simulink library "controllers"  (R2018a)
settings: Solver=VariableStepAuto  StartTime=0.0  StopTime=10.0  RelTol=1e-3
undefined symbols (not defined in the file): ctrl, plant
libraries: controllerComponents x24, simulink x14
settings Model: Creator=mitch  LastModifiedBy=mitch

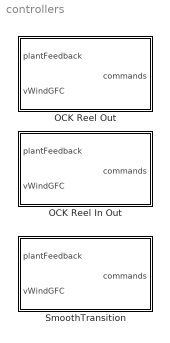
== system controllers ==
  OCK Reel In Out : Subsystem  VariantControl=variantOCKReelInOut
  OCK Reel Out : Subsystem  VariantControl=variantOCK
  SmoothTransition : Subsystem  VariantControl=variantOCKReelInOut

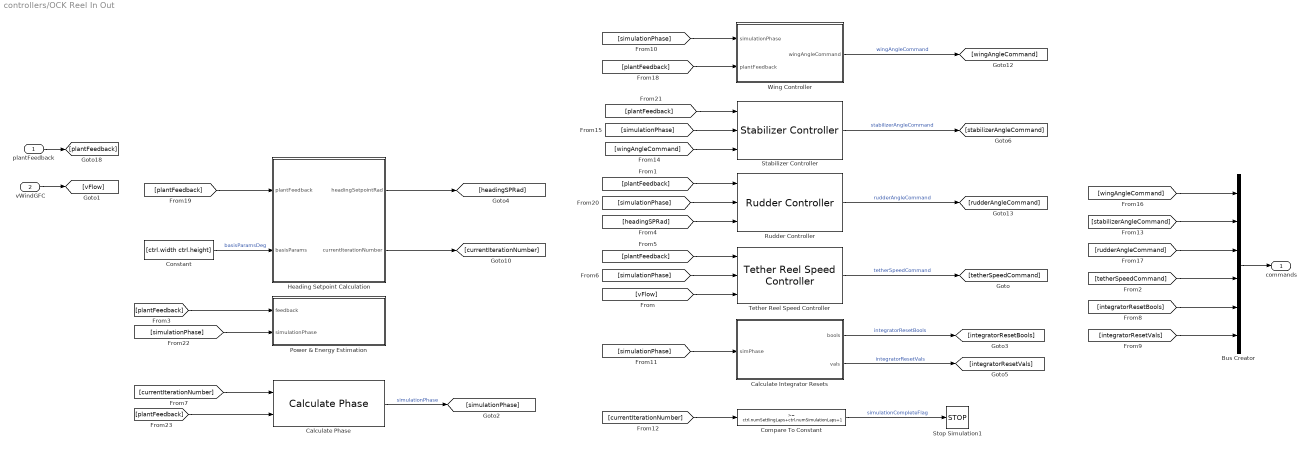
== system controllers/OCK Reel In Out ==
  plantFeedback : Inport  OutDataTypeStr=Bus: busPlantFeedback
  vWindGFC : Inport  Port=2
  Bus Creator : BusCreator  Inputs=6  OutDataTypeStr=Bus: busControllerOutput
  Calculate Integrator Resets : Subsystem
  Calculate Phase : controllerComponents/Calculate Phase
  Compare To Constant : simulink/Logic and Bit Operations/Compare To Constant  relop=>=  const=ctrl.numSettlingLaps+ctrl.numSimulationLaps+1  OutDataTypeStr=boolean
  Constant : Constant  Value=[ctrl.width ctrl.height]
  Heading Setpoint Calculation : Subsystem  VariantControl=variantPureCarrotFollowing
  Power & Energy Estimation : Subsystem
  Rudder Controller : controllerComponents/Rudder Controller
  Stabilizer Controller : controllerComponents/Stabilizer Controller
  Stop Simulation1 : Stop
  Tether Reel Speed Controller : controllerComponents/Tether Reel Speed Controller
  Wing Controller : Subsystem
  commands : Outport  OutDataTypeStr=Bus: busControllerOutput
  wires:
  [plantFeedback] -> Heading Setpoint Calculation/1(plantFeedback)
  Constant/1 -> Heading Setpoint Calculation/2(basisParams)  "basisParamsDeg"
  plantFeedback/1 -> [plantFeedback]
  vWindGFC/1 -> [vFlow]
  Bus Creator/1 -> commands/1
  [currentIterationNumber] -> Compare To Constant/1
  Compare To Constant/1 -> Stop Simulation1/1  "simulationCompleteFlag"
  Heading Setpoint Calculation/2(currentIterationNumber) -> [currentIterationNumber]
  Heading Setpoint Calculation/1(headingSetpointRad) -> [headingSPRad]
  Rudder Controller/1 -> [rudderAngleCommand]  "rudderAngleCommand"
  Tether Reel Speed Controller/1 -> [tetherSpeedCommand]  "tetherSpeedCommand"
  [plantFeedback] -> Power & Energy Estimation/1(feedback)
  [currentIterationNumber] -> Calculate Phase/1
  Calculate Phase/1 -> [simulationPhase]  "simulationPhase"
  [plantFeedback] -> Wing Controller/2(plantFeedback)
  Wing Controller/1(wingAngleCommand) -> [wingAngleCommand]  "wingAngleCommand"
  [simulationPhase] -> Wing Controller/1(simulationPhase)
  [simulationPhase] -> Calculate Integrator Resets/1(simPhase)
  Calculate Integrator Resets/1(bools) -> [integratorResetBools]  "integratorResetBools"
  Calculate Integrator Resets/2(vals) -> [integratorResetVals]  "integratorResetVals"
  [vFlow] -> Tether Reel Speed Controller/3
  [plantFeedback] -> Tether Reel Speed Controller/1
  [simulationPhase] -> Tether Reel Speed Controller/2
  [integratorResetVals] -> Bus Creator/6
  [integratorResetBools] -> Bus Creator/5
  [tetherSpeedCommand] -> Bus Creator/4
  [rudderAngleCommand] -> Bus Creator/3
  [wingAngleCommand] -> Bus Creator/1
  Stabilizer Controller/1 -> [stabilizerAngleCommand]  "stabilizerAngleCommand"
  [stabilizerAngleCommand] -> Bus Creator/2
  [plantFeedback] -> Rudder Controller/1
  [headingSPRad] -> Rudder Controller/3
  [simulationPhase] -> Rudder Controller/2
  [simulationPhase] -> Stabilizer Controller/2
  [plantFeedback] -> Stabilizer Controller/1
  [wingAngleCommand] -> Stabilizer Controller/3
  [simulationPhase] -> Power & Energy Estimation/2(simulationPhase)
  [plantFeedback] -> Calculate Phase/2

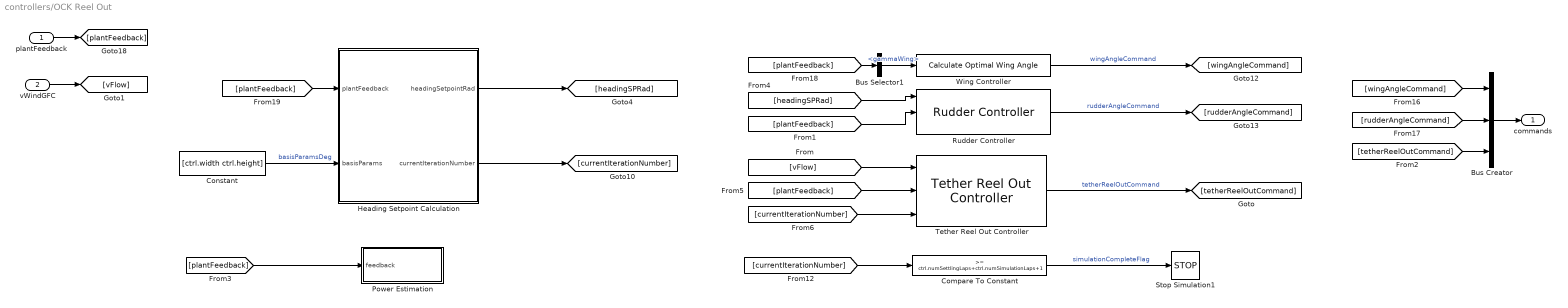
== system controllers/OCK Reel Out ==
  plantFeedback : Inport  OutDataTypeStr=Bus: busPlantFeedback
  vWindGFC : Inport  Port=2
  Bus Creator : BusCreator  Inputs=3  OutDataTypeStr=Bus: busControllerOutput
  Bus Selector1 : BusSelector  OutputSignals=gammaWing
  Compare To Constant : simulink/Logic and Bit Operations/Compare To Constant  relop=>=  const=ctrl.numSettlingLaps+ctrl.numSimulationLaps+1  OutDataTypeStr=boolean
  Constant : Constant  Value=[ctrl.width ctrl.height]
  Heading Setpoint Calculation : Subsystem  VariantControl=variantPureCarrotFollowing
  Power Estimation : Subsystem
  Rudder Controller : controllerComponents/Rudder Controller
  Stop Simulation1 : Stop
  Tether Reel Out Controller : controllerComponents/Tether Reel Out Controller
  Wing Controller : controllerComponents/Calculate Optimal Wing Angle
  commands : Outport  OutDataTypeStr=Bus: busControllerOutput
  wires:
  [plantFeedback] -> Heading Setpoint Calculation/1(plantFeedback)
  Constant/1 -> Heading Setpoint Calculation/2(basisParams)  "basisParamsDeg"
  [plantFeedback] -> Rudder Controller/2
  [plantFeedback] -> Bus Selector1/1
  plantFeedback/1 -> [plantFeedback]
  vWindGFC/1 -> [vFlow]
  Bus Selector1/1 -> Wing Controller/1  "<gammaWing>"
  Bus Creator/1 -> commands/1
  [rudderAngleCommand] -> Bus Creator/2
  [wingAngleCommand] -> Bus Creator/1
  [currentIterationNumber] -> Compare To Constant/1
  Compare To Constant/1 -> Stop Simulation1/1  "simulationCompleteFlag"
  Heading Setpoint Calculation/2(currentIterationNumber) -> [currentIterationNumber]
  Heading Setpoint Calculation/1(headingSetpointRad) -> [headingSPRad]
  [headingSPRad] -> Rudder Controller/1
  Rudder Controller/1 -> [rudderAngleCommand]  "rudderAngleCommand"
  Wing Controller/1 -> [wingAngleCommand]  "wingAngleCommand"
  [tetherReelOutCommand] -> Bus Creator/3
  Tether Reel Out Controller/1 -> [tetherReelOutCommand]  "tetherReelOutCommand"
  [vFlow] -> Tether Reel Out Controller/1
  [plantFeedback] -> Power Estimation/1(feedback)
  [plantFeedback] -> Tether Reel Out Controller/2
  [currentIterationNumber] -> Tether Reel Out Controller/3

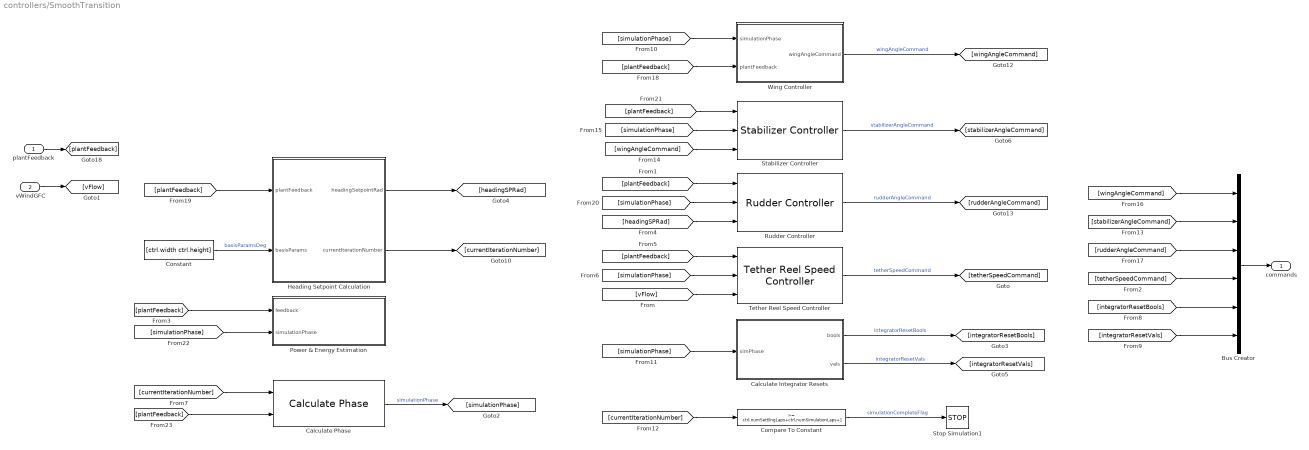
== system controllers/SmoothTransition ==
  plantFeedback : Inport  OutDataTypeStr=Bus: busPlantFeedback
  vWindGFC : Inport  Port=2
  Bus Creator : BusCreator  Inputs=6  OutDataTypeStr=Bus: busControllerOutput
  Calculate Integrator Resets : Subsystem
  Calculate Phase : controllerComponents/Calculate Phase
  Compare To Constant : simulink/Logic and Bit Operations/Compare To Constant  relop=>=  const=ctrl.numSettlingLaps+ctrl.numSimulationLaps+1  OutDataTypeStr=boolean
  Constant : Constant  Value=[ctrl.width ctrl.height]
  Heading Setpoint Calculation : Subsystem  VariantControl=variantPureCarrotFollowing
  Power & Energy Estimation : Subsystem
  Rudder Controller : controllerComponents/Rudder Controller
  Stabilizer Controller : controllerComponents/Stabilizer Controller
  Stop Simulation1 : Stop
  Tether Reel Speed Controller : controllerComponents/Tether Reel Speed Controller
  Wing Controller : Subsystem
  commands : Outport  OutDataTypeStr=Bus: busControllerOutput
  wires:
  [plantFeedback] -> Heading Setpoint Calculation/1(plantFeedback)
  Constant/1 -> Heading Setpoint Calculation/2(basisParams)  "basisParamsDeg"
  plantFeedback/1 -> [plantFeedback]
  vWindGFC/1 -> [vFlow]
  Bus Creator/1 -> commands/1
  [currentIterationNumber] -> Compare To Constant/1
  Compare To Constant/1 -> Stop Simulation1/1  "simulationCompleteFlag"
  Heading Setpoint Calculation/2(currentIterationNumber) -> [currentIterationNumber]
  Heading Setpoint Calculation/1(headingSetpointRad) -> [headingSPRad]
  Rudder Controller/1 -> [rudderAngleCommand]  "rudderAngleCommand"
  Tether Reel Speed Controller/1 -> [tetherSpeedCommand]  "tetherSpeedCommand"
  [plantFeedback] -> Power & Energy Estimation/1(feedback)
  [currentIterationNumber] -> Calculate Phase/1
  Calculate Phase/1 -> [simulationPhase]  "simulationPhase"
  [plantFeedback] -> Wing Controller/2(plantFeedback)
  Wing Controller/1(wingAngleCommand) -> [wingAngleCommand]  "wingAngleCommand"
  [simulationPhase] -> Wing Controller/1(simulationPhase)
  [simulationPhase] -> Calculate Integrator Resets/1(simPhase)
  Calculate Integrator Resets/1(bools) -> [integratorResetBools]  "integratorResetBools"
  Calculate Integrator Resets/2(vals) -> [integratorResetVals]  "integratorResetVals"
  [vFlow] -> Tether Reel Speed Controller/3
  [plantFeedback] -> Tether Reel Speed Controller/1
  [simulationPhase] -> Tether Reel Speed Controller/2
  [integratorResetVals] -> Bus Creator/6
  [integratorResetBools] -> Bus Creator/5
  [tetherSpeedCommand] -> Bus Creator/4
  [rudderAngleCommand] -> Bus Creator/3
  [wingAngleCommand] -> Bus Creator/1
  Stabilizer Controller/1 -> [stabilizerAngleCommand]  "stabilizerAngleCommand"
  [stabilizerAngleCommand] -> Bus Creator/2
  [plantFeedback] -> Rudder Controller/1
  [headingSPRad] -> Rudder Controller/3
  [simulationPhase] -> Rudder Controller/2
  [simulationPhase] -> Stabilizer Controller/2
  [plantFeedback] -> Stabilizer Controller/1
  [wingAngleCommand] -> Stabilizer Controller/3
  [simulationPhase] -> Power & Energy Estimation/2(simulationPhase)
  [plantFeedback] -> Calculate Phase/2

== system controllers/OCK Reel In Out/Calculate Integrator Resets ==
  simPhase : Inport
  Calculate Booleans : Subsystem
  Calculate Values : Subsystem
  Compare To Constant : simulink/Logic and Bit Operations/Compare To Constant  relop===  const=2  OutDataTypeStr=boolean
  Delay : Delay  DelayLength=1  InitialCondition=0
  bools : Outport
  vals : Outport  Port=2
  wires:
  simPhase/1 -> Delay/1
  Calculate Booleans/1(bools) -> bools/1
  Calculate Values/1(bools) -> vals/1
  Compare To Constant/1 -> Calculate Booleans/1(reelInFlag), Calculate Values/1(reelInFlag)
  Delay/1 -> Compare To Constant/1

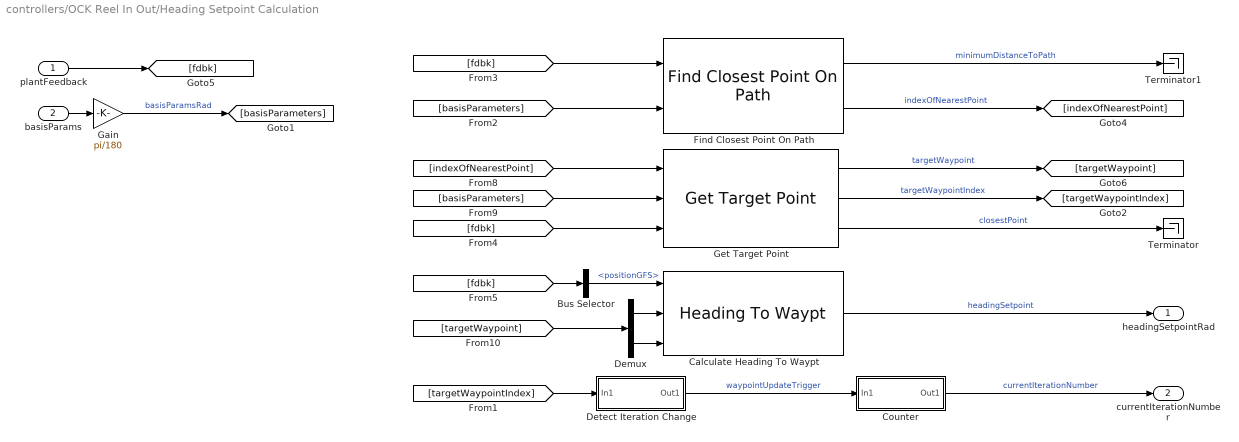
== system controllers/OCK Reel In Out/Heading Setpoint Calculation ==
  plantFeedback : Inport  OutDataTypeStr=Bus: busPlantFeedback
  basisParams : Inport  Port=2
  Bus Selector : BusSelector  OutputSignals=positionGFS
  Calculate Heading To Waypt : controllerComponents/Heading To Waypt
  Counter : Subsystem
  Demux : Demux  Outputs=2
  Detect Iteration Change : Subsystem
  Find Closest Point On Path : controllerComponents/Find Closest Point On Path
  Gain : Gain  Gain=pi/180
  Get Target Point : controllerComponents/Get Target Point
  Terminator : Terminator
  Terminator1 : Terminator
  headingSetpointRad : Outport
  currentIterationNumber : Outport  Port=2
  wires:
  Get Target Point/3 -> Terminator/1  "closestPoint"
  plantFeedback/1 -> [fdbk]
  Get Target Point/2 -> [targetWaypointIndex]  "targetWaypointIndex"
  Detect Iteration Change/1(Out1) -> Counter/1(In1)  "waypointUpdateTrigger"
  Counter/1(Out1) -> currentIterationNumber/1  "currentIterationNumber"
  [targetWaypointIndex] -> Detect Iteration Change/1(In1)
  Calculate Heading To Waypt/1 -> headingSetpointRad/1  "headingSetpoint"
  [targetWaypoint] -> Demux/1
  Get Target Point/1 -> [targetWaypoint]  "targetWaypoint"
  [basisParameters] -> Get Target Point/2
  [indexOfNearestPoint] -> Get Target Point/1
  Find Closest Point On Path/2 -> [indexOfNearestPoint]  "indexOfNearestPoint"
  Find Closest Point On Path/1 -> Terminator1/1  "minimumDistanceToPath"
  Demux/2 -> Calculate Heading To Waypt/3
  Demux/1 -> Calculate Heading To Waypt/2
  [basisParameters] -> Find Closest Point On Path/2
  [fdbk] -> Find Closest Point On Path/1
  [fdbk] -> Get Target Point/3
  basisParams/1 -> Gain/1
  [fdbk] -> Bus Selector/1
  Bus Selector/1 -> Calculate Heading To Waypt/1  "<positionGFS>"
  Gain/1 -> [basisParameters]  "basisParamsRad"

== system controllers/OCK Reel In Out/Power & Energy Estimation ==
  feedback : Inport
  simulationPhase : Inport  Port=2
  Bus Selector : BusSelector  OutputSignals=rDot,tetherTension
  Compare To Constant : simulink/Logic and Bit Operations/Compare To Constant  relop=>=  const=1  OutDataTypeStr=boolean
  Constant : Constant  Value=0
  Integrator : Integrator  ExternalReset=rising  InitialConditionSource=external
  Product : Product
  Terminator : Terminator
  Terminator1 : Terminator
  wires:
  Product/1 -> Integrator/1, Terminator/1  "powerEstimate"
  feedback/1 -> Bus Selector/1
  Bus Selector/1 -> Product/1  "<rDot>"
  Bus Selector/2 -> Product/2  "<tetherTension>"
  Integrator/1 -> Terminator1/1  "netEnergy"
  simulationPhase/1 -> Compare To Constant/1
  Compare To Constant/1 -> Integrator/2
  Constant/1 -> Integrator/3

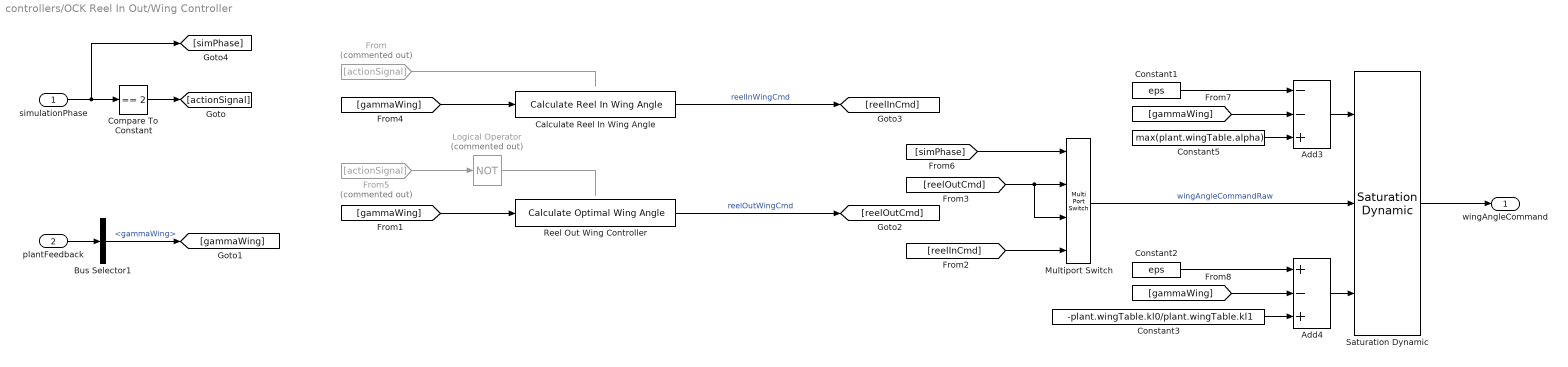
== system controllers/OCK Reel In Out/Wing Controller ==
  simulationPhase : Inport
  plantFeedback : Inport  Port=2
  Add3 : Sum  Inputs=--+
  Add4 : Sum  Inputs=+-+
  Bus Selector1 : BusSelector  OutputSignals=gammaWing
  Calculate Reel In Wing Angle : controllerComponents/Calculate Reel In Wing Angle
  Compare To Constant : simulink/Logic and Bit Operations/Compare To Constant  relop===  const=2  OutDataTypeStr=boolean
  Constant1 : Constant  Value=eps
  Constant2 : Constant  Value=eps
  Constant3 : Constant  Value=-plant.wingTable.kl0/plant.wingTable.kl1
  Constant5 : Constant  Value=max(plant.wingTable.alpha)
  From : From  Commented=on  GotoTag=actionSignal
  From5 : From  Commented=on  GotoTag=actionSignal
  Logical Operator : Logic  Commented=on  Operator=NOT  AllPortsSameDT=off  OutDataTypeStr=boolean
  Multiport Switch : MultiPortSwitch  DataPortOrder=Zero-based contiguous  zeroidx=on
  Reel Out Wing Controller : controllerComponents/Calculate Optimal Wing Angle
  Saturation Dynamic : simulink/Discontinuities/Saturation Dynamic  OutMin=[]  OutMax=[]  OutDataTypeStr=Inherit: Same as second input  OutDataType=fixdt(1, 16)  OutScaling=2^-10  DoSatur=off
  wingAngleCommand : Outport
  wires:
  plantFeedback/1 -> Bus Selector1/1
  simulationPhase/1 -> [simPhase], Compare To Constant/1
  Add4/1 -> Saturation Dynamic/3
  Add3/1 -> Saturation Dynamic/1
  Saturation Dynamic/1 -> wingAngleCommand/1
  Bus Selector1/1 -> [gammaWing]  "<gammaWing>"
  [gammaWing] -> Reel Out Wing Controller/1
  Reel Out Wing Controller/1 -> [reelOutCmd]  "reelOutWingCmd"
  Calculate Reel In Wing Angle/1 -> [reelInCmd]  "reelInWingCmd"
  [gammaWing] -> Calculate Reel In Wing Angle/1
  Logical Operator/1 -> ?
  Compare To Constant/1 -> [actionSignal]
  From/1 -> ?
  From5/1 -> Logical Operator/1
  Constant5/1 -> Add3/3
  Constant1/1 -> Add3/1
  [gammaWing] -> Add3/2
  Constant3/1 -> Add4/3
  [gammaWing] -> Add4/2
  Constant2/1 -> Add4/1
  Multiport Switch/1 -> Saturation Dynamic/2  "wingAngleCommandRaw"
  [simPhase] -> Multiport Switch/1
  [reelOutCmd] -> Multiport Switch/3, Multiport Switch/2
  [reelInCmd] -> Multiport Switch/4

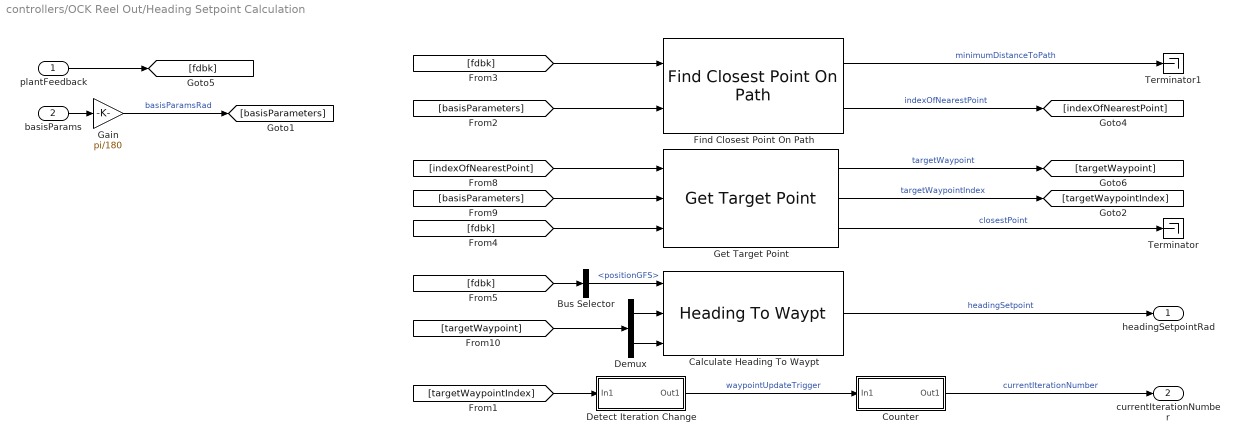
== system controllers/OCK Reel Out/Heading Setpoint Calculation ==
  plantFeedback : Inport  OutDataTypeStr=Bus: busPlantFeedback
  basisParams : Inport  Port=2
  Bus Selector : BusSelector  OutputSignals=positionGFS
  Calculate Heading To Waypt : controllerComponents/Heading To Waypt
  Counter : Subsystem
  Demux : Demux  Outputs=2
  Detect Iteration Change : Subsystem
  Find Closest Point On Path : controllerComponents/Find Closest Point On Path
  Gain : Gain  Gain=pi/180
  Get Target Point : controllerComponents/Get Target Point
  Terminator : Terminator
  Terminator1 : Terminator
  headingSetpointRad : Outport
  currentIterationNumber : Outport  Port=2
  wires:
  Get Target Point/3 -> Terminator/1  "closestPoint"
  plantFeedback/1 -> [fdbk]
  Get Target Point/2 -> [targetWaypointIndex]  "targetWaypointIndex"
  Detect Iteration Change/1(Out1) -> Counter/1(In1)  "waypointUpdateTrigger"
  Counter/1(Out1) -> currentIterationNumber/1  "currentIterationNumber"
  [targetWaypointIndex] -> Detect Iteration Change/1(In1)
  Calculate Heading To Waypt/1 -> headingSetpointRad/1  "headingSetpoint"
  [targetWaypoint] -> Demux/1
  Get Target Point/1 -> [targetWaypoint]  "targetWaypoint"
  [basisParameters] -> Get Target Point/2
  [indexOfNearestPoint] -> Get Target Point/1
  Find Closest Point On Path/2 -> [indexOfNearestPoint]  "indexOfNearestPoint"
  Find Closest Point On Path/1 -> Terminator1/1  "minimumDistanceToPath"
  Demux/2 -> Calculate Heading To Waypt/3
  Demux/1 -> Calculate Heading To Waypt/2
  [basisParameters] -> Find Closest Point On Path/2
  [fdbk] -> Find Closest Point On Path/1
  [fdbk] -> Get Target Point/3
  basisParams/1 -> Gain/1
  [fdbk] -> Bus Selector/1
  Bus Selector/1 -> Calculate Heading To Waypt/1  "<positionGFS>"
  Gain/1 -> [basisParameters]  "basisParamsRad"

== system controllers/OCK Reel Out/Power Estimation ==
  feedback : Inport
  Bus Selector : BusSelector  OutputSignals=rDot,tetherTension
  Product : Product
  Terminator : Terminator
  wires:
  Product/1 -> Terminator/1  "powerEstimate"
  feedback/1 -> Bus Selector/1
  Bus Selector/1 -> Product/1  "<rDot>"
  Bus Selector/2 -> Product/2  "<tetherTension>"

== system controllers/SmoothTransition/Calculate Integrator Resets ==
  simPhase : Inport
  Calculate Booleans : Subsystem
  Calculate Values : Subsystem
  Compare To Constant : simulink/Logic and Bit Operations/Compare To Constant  relop===  const=2  OutDataTypeStr=boolean
  Delay : Delay  DelayLength=1  InitialCondition=0
  bools : Outport
  vals : Outport  Port=2
  wires:
  simPhase/1 -> Delay/1
  Calculate Booleans/1(bools) -> bools/1
  Calculate Values/1(bools) -> vals/1
  Compare To Constant/1 -> Calculate Booleans/1(reelInFlag), Calculate Values/1(reelInFlag)
  Delay/1 -> Compare To Constant/1

== system controllers/SmoothTransition/Heading Setpoint Calculation ==
  plantFeedback : Inport  OutDataTypeStr=Bus: busPlantFeedback
  basisParams : Inport  Port=2
  Bus Selector : BusSelector  OutputSignals=positionGFS
  Calculate Heading To Waypt : controllerComponents/Heading To Waypt
  Counter : Subsystem
  Demux : Demux  Outputs=2
  Detect Iteration Change : Subsystem
  Find Closest Point On Path : controllerComponents/Find Closest Point On Path
  Gain : Gain  Gain=pi/180
  Get Target Point : controllerComponents/Get Target Point
  Terminator : Terminator
  Terminator1 : Terminator
  headingSetpointRad : Outport
  currentIterationNumber : Outport  Port=2
  wires:
  Get Target Point/3 -> Terminator/1  "closestPoint"
  plantFeedback/1 -> [fdbk]
  Get Target Point/2 -> [targetWaypointIndex]  "targetWaypointIndex"
  Detect Iteration Change/1(Out1) -> Counter/1(In1)  "waypointUpdateTrigger"
  Counter/1(Out1) -> currentIterationNumber/1  "currentIterationNumber"
  [targetWaypointIndex] -> Detect Iteration Change/1(In1)
  Calculate Heading To Waypt/1 -> headingSetpointRad/1  "headingSetpoint"
  [targetWaypoint] -> Demux/1
  Get Target Point/1 -> [targetWaypoint]  "targetWaypoint"
  [basisParameters] -> Get Target Point/2
  [indexOfNearestPoint] -> Get Target Point/1
  Find Closest Point On Path/2 -> [indexOfNearestPoint]  "indexOfNearestPoint"
  Find Closest Point On Path/1 -> Terminator1/1  "minimumDistanceToPath"
  Demux/2 -> Calculate Heading To Waypt/3
  Demux/1 -> Calculate Heading To Waypt/2
  [basisParameters] -> Find Closest Point On Path/2
  [fdbk] -> Find Closest Point On Path/1
  [fdbk] -> Get Target Point/3
  basisParams/1 -> Gain/1
  [fdbk] -> Bus Selector/1
  Bus Selector/1 -> Calculate Heading To Waypt/1  "<positionGFS>"
  Gain/1 -> [basisParameters]  "basisParamsRad"

== system controllers/SmoothTransition/Power & Energy Estimation ==
  feedback : Inport
  simulationPhase : Inport  Port=2
  Bus Selector : BusSelector  OutputSignals=rDot,tetherTension
  Compare To Constant : simulink/Logic and Bit Operations/Compare To Constant  relop=>=  const=1  OutDataTypeStr=boolean
  Constant : Constant  Value=0
  Integrator : Integrator  ExternalReset=rising  InitialConditionSource=external
  Product : Product
  Terminator : Terminator
  Terminator1 : Terminator
  wires:
  Product/1 -> Integrator/1, Terminator/1  "powerEstimate"
  feedback/1 -> Bus Selector/1
  Bus Selector/1 -> Product/1  "<rDot>"
  Bus Selector/2 -> Product/2  "<tetherTension>"
  Integrator/1 -> Terminator1/1  "netEnergy"
  simulationPhase/1 -> Compare To Constant/1
  Compare To Constant/1 -> Integrator/2
  Constant/1 -> Integrator/3

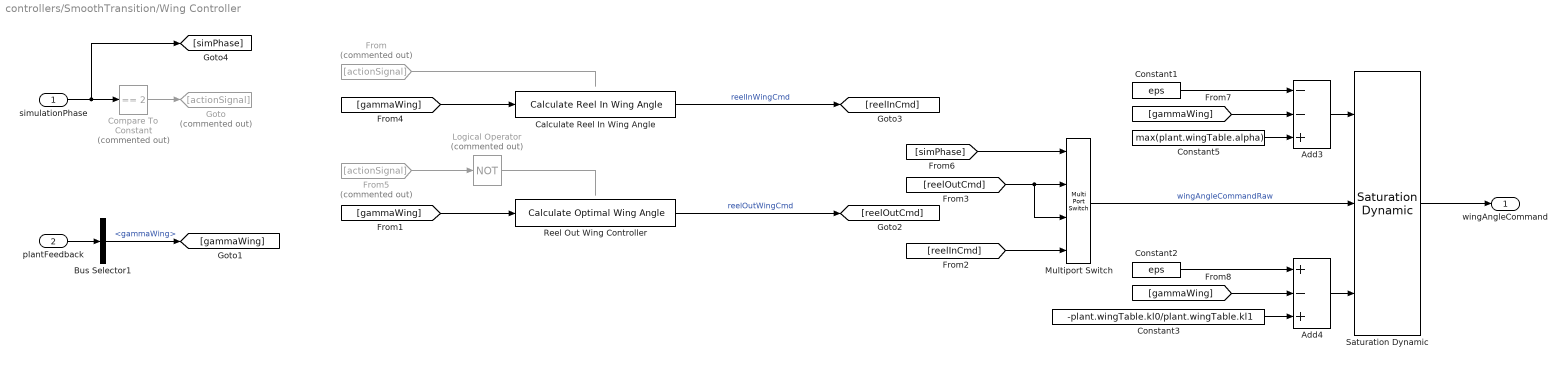
== system controllers/SmoothTransition/Wing Controller ==
  simulationPhase : Inport
  plantFeedback : Inport  Port=2
  Add3 : Sum  Inputs=--+
  Add4 : Sum  Inputs=+-+
  Bus Selector1 : BusSelector  OutputSignals=gammaWing
  Calculate Reel In Wing Angle : controllerComponents/Calculate Reel In Wing Angle
  Compare To Constant : simulink/Logic and Bit Operations/Compare To Constant  Commented=on  relop===  const=2  OutDataTypeStr=boolean
  Constant1 : Constant  Value=eps
  Constant2 : Constant  Value=eps
  Constant3 : Constant  Value=-plant.wingTable.kl0/plant.wingTable.kl1
  Constant5 : Constant  Value=max(plant.wingTable.alpha)
  From : From  Commented=on  GotoTag=actionSignal
  From5 : From  Commented=on  GotoTag=actionSignal
  Goto : Goto  Commented=on  GotoTag=actionSignal
  Logical Operator : Logic  Commented=on  Operator=NOT  AllPortsSameDT=off  OutDataTypeStr=boolean
  Multiport Switch : MultiPortSwitch  DataPortOrder=Zero-based contiguous  zeroidx=on
  Reel Out Wing Controller : controllerComponents/Calculate Optimal Wing Angle
  Saturation Dynamic : simulink/Discontinuities/Saturation Dynamic  OutMin=[]  OutMax=[]  OutDataTypeStr=Inherit: Same as second input  OutDataType=fixdt(1, 16)  OutScaling=2^-10  DoSatur=off
  wingAngleCommand : Outport
  wires:
  plantFeedback/1 -> Bus Selector1/1
  simulationPhase/1 -> [simPhase], Compare To Constant/1
  Add4/1 -> Saturation Dynamic/3
  Add3/1 -> Saturation Dynamic/1
  Saturation Dynamic/1 -> wingAngleCommand/1
  Bus Selector1/1 -> [gammaWing]  "<gammaWing>"
  [gammaWing] -> Reel Out Wing Controller/1
  Reel Out Wing Controller/1 -> [reelOutCmd]  "reelOutWingCmd"
  Calculate Reel In Wing Angle/1 -> [reelInCmd]  "reelInWingCmd"
  [gammaWing] -> Calculate Reel In Wing Angle/1
  Logical Operator/1 -> ?
  Compare To Constant/1 -> Goto/1
  From/1 -> ?
  From5/1 -> Logical Operator/1
  Constant5/1 -> Add3/3
  Constant1/1 -> Add3/1
  [gammaWing] -> Add3/2
  Constant3/1 -> Add4/3
  [gammaWing] -> Add4/2
  Constant2/1 -> Add4/1
  Multiport Switch/1 -> Saturation Dynamic/2  "wingAngleCommandRaw"
  [simPhase] -> Multiport Switch/1
  [reelOutCmd] -> Multiport Switch/3, Multiport Switch/2
  [reelInCmd] -> Multiport Switch/4

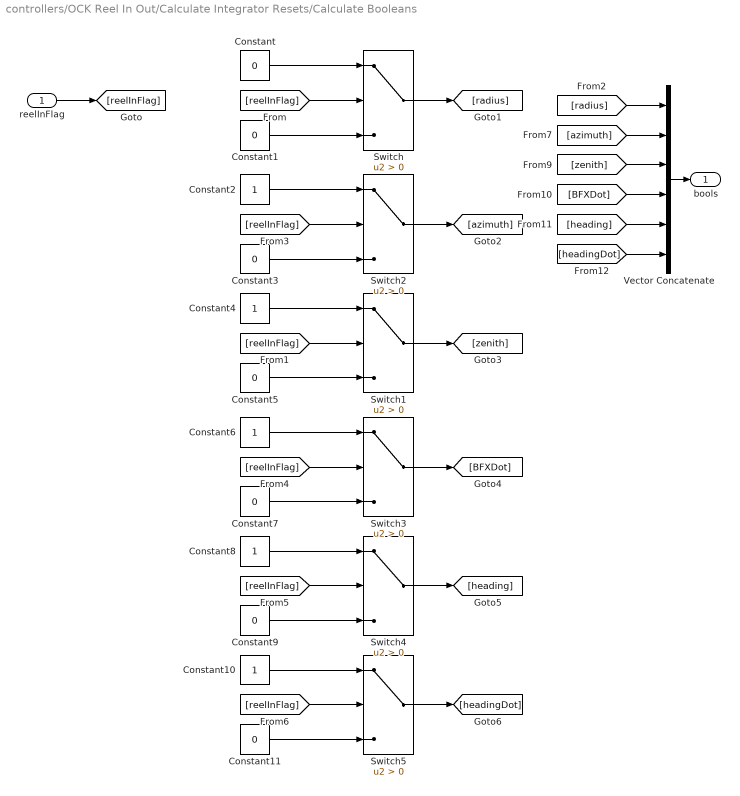
== system controllers/OCK Reel In Out/Calculate Integrator Resets/Calculate Booleans ==
  reelInFlag : Inport
  Constant{,1,3,5,7,9,11} (7 alike) : Constant  Value=0  OutDataTypeStr=boolean
  Constant{2,4,6,8,10} (5 alike) : Constant  OutDataTypeStr=boolean
  Switch{,1..5} (6 alike) : Switch  Criteria=u2 > Threshold
  Vector Concatenate : Concatenate  NumInputs=6
  bools : Outport
  wires:
  Constant8/1 -> Switch4/1
  Switch4/1 -> [heading]
  Constant9/1 -> Switch4/3
  [reelInFlag] -> Switch4/2
  Constant5/1 -> Switch1/3
  Constant4/1 -> Switch1/1
  [reelInFlag] -> Switch1/2
  [reelInFlag] -> Switch/2
  Switch1/1 -> [zenith]
  [radius] -> Vector Concatenate/1
  [reelInFlag] -> Switch5/2
  Switch5/1 -> [headingDot]
  Constant10/1 -> Switch5/1
  Constant11/1 -> Switch5/3
  Constant/1 -> Switch/1
  [BFXDot] -> Vector Concatenate/4
  Switch/1 -> [radius]
  Constant1/1 -> Switch/3
  Constant7/1 -> Switch3/3
  [reelInFlag] -> Switch3/2
  Constant6/1 -> Switch3/1
  Switch3/1 -> [BFXDot]
  Vector Concatenate/1 -> bools/1
  [azimuth] -> Vector Concatenate/2
  [zenith] -> Vector Concatenate/3
  [heading] -> Vector Concatenate/5
  Constant2/1 -> Switch2/1
  Constant3/1 -> Switch2/3
  Switch2/1 -> [azimuth]
  [reelInFlag] -> Switch2/2
  [headingDot] -> Vector Concatenate/6
  reelInFlag/1 -> [reelInFlag]

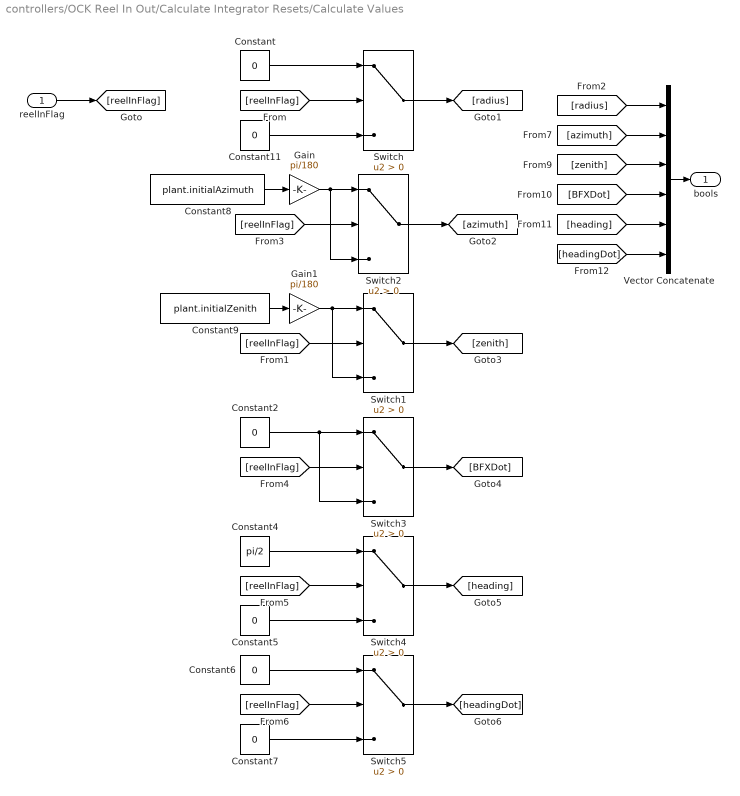
== system controllers/OCK Reel In Out/Calculate Integrator Resets/Calculate Values ==
  reelInFlag : Inport
  Constant{,2,5..7,11} (6 alike) : Constant  Value=0  OutDataTypeStr=double
  Constant4 : Constant  Value=pi/2  OutDataTypeStr=double
  Constant8 : Constant  Value=plant.initialAzimuth  OutDataTypeStr=double
  Constant9 : Constant  Value=plant.initialZenith  OutDataTypeStr=double
  Gain : Gain  Gain=pi/180
  Gain1 : Gain  Gain=pi/180
  Switch{,1..5} (6 alike) : Switch  Criteria=u2 > Threshold
  Vector Concatenate : Concatenate  NumInputs=6
  bools : Outport
  wires:
  Constant4/1 -> Switch4/1
  Switch4/1 -> [heading]
  Constant5/1 -> Switch4/3
  [reelInFlag] -> Switch4/2
  Gain1/1 -> Switch1/3, Switch1/1
  Constant9/1 -> Gain1/1
  [reelInFlag] -> Switch1/2
  [reelInFlag] -> Switch/2
  Switch1/1 -> [zenith]
  [radius] -> Vector Concatenate/1
  [reelInFlag] -> Switch5/2
  Switch5/1 -> [headingDot]
  Constant6/1 -> Switch5/1
  Constant7/1 -> Switch5/3
  Constant/1 -> Switch/1
  [BFXDot] -> Vector Concatenate/4
  Switch/1 -> [radius]
  Constant11/1 -> Switch/3
  Constant2/1 -> Switch3/3, Switch3/1
  [reelInFlag] -> Switch3/2
  Switch3/1 -> [BFXDot]
  Vector Concatenate/1 -> bools/1
  [azimuth] -> Vector Concatenate/2
  [zenith] -> Vector Concatenate/3
  [heading] -> Vector Concatenate/5
  Constant8/1 -> Gain/1
  Gain/1 -> Switch2/3, Switch2/1
  Switch2/1 -> [azimuth]
  [reelInFlag] -> Switch2/2
  [headingDot] -> Vector Concatenate/6
  reelInFlag/1 -> [reelInFlag]

== system controllers/OCK Reel In Out/Heading Setpoint Calculation/Counter ==
  In1 : Inport
  Add : Sum
  Data Type Conversion : DataTypeConversion  OutDataTypeStr=uint8
  Memory : Memory  InitialCondition=1
  Out1 : Outport  OutDataTypeStr=double
  wires:
  Data Type Conversion/1 -> Add/1
  In1/1 -> Data Type Conversion/1
  Memory/1 -> Add/2
  Add/1 -> Memory/1, Out1/1

== system controllers/OCK Reel In Out/Heading Setpoint Calculation/Detect Iteration Change ==
  In1 : Inport
  Detect Decrease : simulink/Logic and Bit Operations/Detect Decrease  vinit=0.0  OutDataTypeStr=boolean
  Out1 : Outport
  wires:
  Detect Decrease/1 -> Out1/1
  In1/1 -> Detect Decrease/1

== system controllers/OCK Reel Out/Heading Setpoint Calculation/Counter ==
  In1 : Inport
  Add : Sum
  Data Type Conversion : DataTypeConversion  OutDataTypeStr=uint8
  Memory : Memory  InitialCondition=1
  Out1 : Outport  OutDataTypeStr=double
  wires:
  Data Type Conversion/1 -> Add/1
  In1/1 -> Data Type Conversion/1
  Memory/1 -> Add/2
  Add/1 -> Memory/1, Out1/1

== system controllers/OCK Reel Out/Heading Setpoint Calculation/Detect Iteration Change ==
  In1 : Inport
  Detect Decrease : simulink/Logic and Bit Operations/Detect Decrease  vinit=0.0  OutDataTypeStr=boolean
  Out1 : Outport
  wires:
  Detect Decrease/1 -> Out1/1
  In1/1 -> Detect Decrease/1

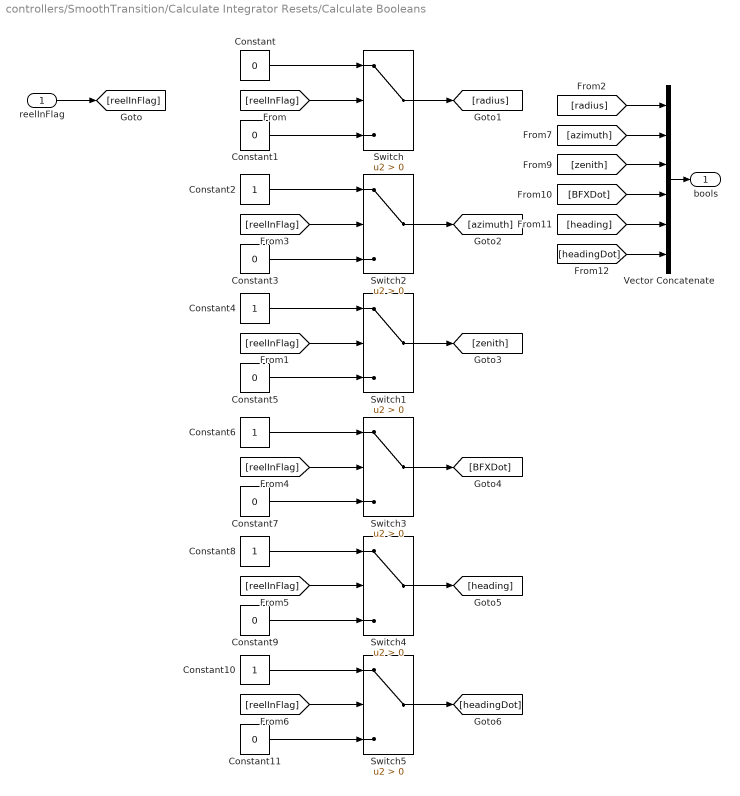
== system controllers/SmoothTransition/Calculate Integrator Resets/Calculate Booleans ==
  reelInFlag : Inport
  Constant{,1,3,5,7,9,11} (7 alike) : Constant  Value=0  OutDataTypeStr=boolean
  Constant{2,4,6,8,10} (5 alike) : Constant  OutDataTypeStr=boolean
  Switch{,1..5} (6 alike) : Switch  Criteria=u2 > Threshold
  Vector Concatenate : Concatenate  NumInputs=6
  bools : Outport
  wires:
  Constant8/1 -> Switch4/1
  Switch4/1 -> [heading]
  Constant9/1 -> Switch4/3
  [reelInFlag] -> Switch4/2
  Constant5/1 -> Switch1/3
  Constant4/1 -> Switch1/1
  [reelInFlag] -> Switch1/2
  [reelInFlag] -> Switch/2
  Switch1/1 -> [zenith]
  [radius] -> Vector Concatenate/1
  [reelInFlag] -> Switch5/2
  Switch5/1 -> [headingDot]
  Constant10/1 -> Switch5/1
  Constant11/1 -> Switch5/3
  Constant/1 -> Switch/1
  [BFXDot] -> Vector Concatenate/4
  Switch/1 -> [radius]
  Constant1/1 -> Switch/3
  Constant7/1 -> Switch3/3
  [reelInFlag] -> Switch3/2
  Constant6/1 -> Switch3/1
  Switch3/1 -> [BFXDot]
  Vector Concatenate/1 -> bools/1
  [azimuth] -> Vector Concatenate/2
  [zenith] -> Vector Concatenate/3
  [heading] -> Vector Concatenate/5
  Constant2/1 -> Switch2/1
  Constant3/1 -> Switch2/3
  Switch2/1 -> [azimuth]
  [reelInFlag] -> Switch2/2
  [headingDot] -> Vector Concatenate/6
  reelInFlag/1 -> [reelInFlag]

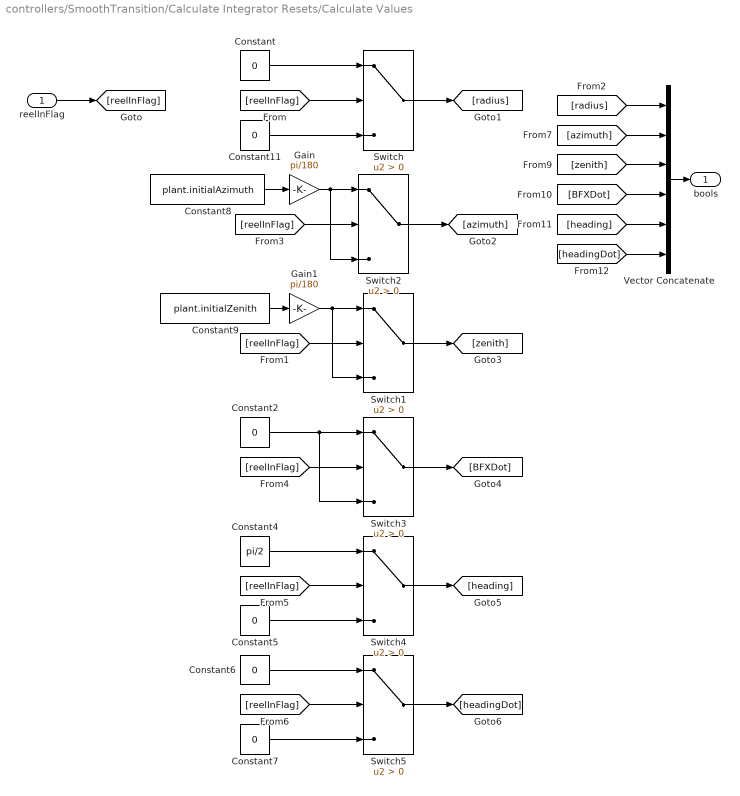
== system controllers/SmoothTransition/Calculate Integrator Resets/Calculate Values ==
  reelInFlag : Inport
  Constant{,2,5..7,11} (6 alike) : Constant  Value=0  OutDataTypeStr=double
  Constant4 : Constant  Value=pi/2  OutDataTypeStr=double
  Constant8 : Constant  Value=plant.initialAzimuth  OutDataTypeStr=double
  Constant9 : Constant  Value=plant.initialZenith  OutDataTypeStr=double
  Gain : Gain  Gain=pi/180
  Gain1 : Gain  Gain=pi/180
  Switch{,1..5} (6 alike) : Switch  Criteria=u2 > Threshold
  Vector Concatenate : Concatenate  NumInputs=6
  bools : Outport
  wires:
  Constant4/1 -> Switch4/1
  Switch4/1 -> [heading]
  Constant5/1 -> Switch4/3
  [reelInFlag] -> Switch4/2
  Gain1/1 -> Switch1/3, Switch1/1
  Constant9/1 -> Gain1/1
  [reelInFlag] -> Switch1/2
  [reelInFlag] -> Switch/2
  Switch1/1 -> [zenith]
  [radius] -> Vector Concatenate/1
  [reelInFlag] -> Switch5/2
  Switch5/1 -> [headingDot]
  Constant6/1 -> Switch5/1
  Constant7/1 -> Switch5/3
  Constant/1 -> Switch/1
  [BFXDot] -> Vector Concatenate/4
  Switch/1 -> [radius]
  Constant11/1 -> Switch/3
  Constant2/1 -> Switch3/3, Switch3/1
  [reelInFlag] -> Switch3/2
  Switch3/1 -> [BFXDot]
  Vector Concatenate/1 -> bools/1
  [azimuth] -> Vector Concatenate/2
  [zenith] -> Vector Concatenate/3
  [heading] -> Vector Concatenate/5
  Constant8/1 -> Gain/1
  Gain/1 -> Switch2/3, Switch2/1
  Switch2/1 -> [azimuth]
  [reelInFlag] -> Switch2/2
  [headingDot] -> Vector Concatenate/6
  reelInFlag/1 -> [reelInFlag]

== system controllers/SmoothTransition/Heading Setpoint Calculation/Counter ==
  In1 : Inport
  Add : Sum
  Data Type Conversion : DataTypeConversion  OutDataTypeStr=uint8
  Memory : Memory  InitialCondition=1
  Out1 : Outport  OutDataTypeStr=double
  wires:
  Data Type Conversion/1 -> Add/1
  In1/1 -> Data Type Conversion/1
  Memory/1 -> Add/2
  Add/1 -> Memory/1, Out1/1

== system controllers/SmoothTransition/Heading Setpoint Calculation/Detect Iteration Change ==
  In1 : Inport
  Detect Decrease : simulink/Logic and Bit Operations/Detect Decrease  vinit=0.0  OutDataTypeStr=boolean
  Out1 : Outport
  wires:
  Detect Decrease/1 -> Out1/1
  In1/1 -> Detect Decrease/1
